simulink model "AssembledTEST1"  (R2016b)
settings: Solver=VariableStepAuto  StartTime=0.0  StopTime=60  RelTol=1e-9
values from neighbouring files (symbols this model uses):
  DOWN_0 = -xtrim(12)    [Comparison_NonLin.m]    (also in InitialiseJ31.m = 1830.0192; Trim.m)
  EAST_0 = xtrim(11)    [Comparison_NonLin.m]    (also in InitialiseJ31.m = 0; Trim.m)
  FLAP = 0    [InitialiseJ31.m]
  INERTIA = [IXX,IXY,IXZ;IXY,IYY,IYZ;IXZ,IYZ,IZZ]    [InitialiseJ31.m]
  NORTH_0 = xtrim(10)    [Comparison_NonLin.m]    (also in InitialiseJ31.m = 0; Trim.m)
  P_0 = xtrim(4)    [Comparison_NonLin.m]    (also in InitialiseJ31.m = 0; Trim.m)
  PHI_0 = xtrim(7)    [Comparison_NonLin.m]    (also in Trim.m)
  PSI_0 = xtrim(9)    [Comparison_NonLin.m]    (also in Trim.m)
  Q_0 = xtrim(5)    [Comparison_NonLin.m]    (also in InitialiseJ31.m = 0; Trim.m)
  R2D = 180/pi    (= 57.2957795131)    [InitialiseJ31.m]
  R_0 = xtrim(6)    [Comparison_NonLin.m]    (also in InitialiseJ31.m = 0; Trim.m)
  THETA_0 = xtrim(8)    [Comparison_NonLin.m]    (also in Trim.m)
  U_0 = xtrim(1)    [Comparison_NonLin.m]    (also in Trim.m)
  V_0 = xtrim(2)    [Comparison_NonLin.m]    (also in Trim.m)
  W_0 = xtrim(3)    [Comparison_NonLin.m]    (also in Trim.m)
undefined symbols (not defined in the file or in its folder): ail_data, Ap, Aw, b, beta0_data, c0, c_i, cdrag_data, CG, clean_wing_data, crt, CT_data, D, D0q_10, D0q_20, D0q_35, DCDi_data, DCM0b, Deh_f_on_data, Deh_on_data, df, Dqhq_data, e0, e_data10, e_data20, e_data35, elaw_0, elaw_1, elaw_2, flaps_lift_data, flaps_moment_data, flaps_tail_data, flaps_wing_data, fmc_data, fmf_data, fmn_data, fus_data, gamma_t, h_data10, h_data20, h_data35, it, iw, Iwn2, J_W, K1_data, k1f_data, k_data, L_r0_10f, L_r0_20f, L_r0_35f, l_t, ld_data, Lt, Lt_dash, Lv_b, Lv_h, Lv_n, mac, mach_ffr ... (+39)
libraries: aerolibasang x3, aerolibatmos2 x1
(part 1 of 5)
settings Model: Creator=pereantoni  LastModifiedBy=carles
settings SolverCC: ZeroCrossControl=DisableAll
settings DataIOCC: SaveFormat=Array

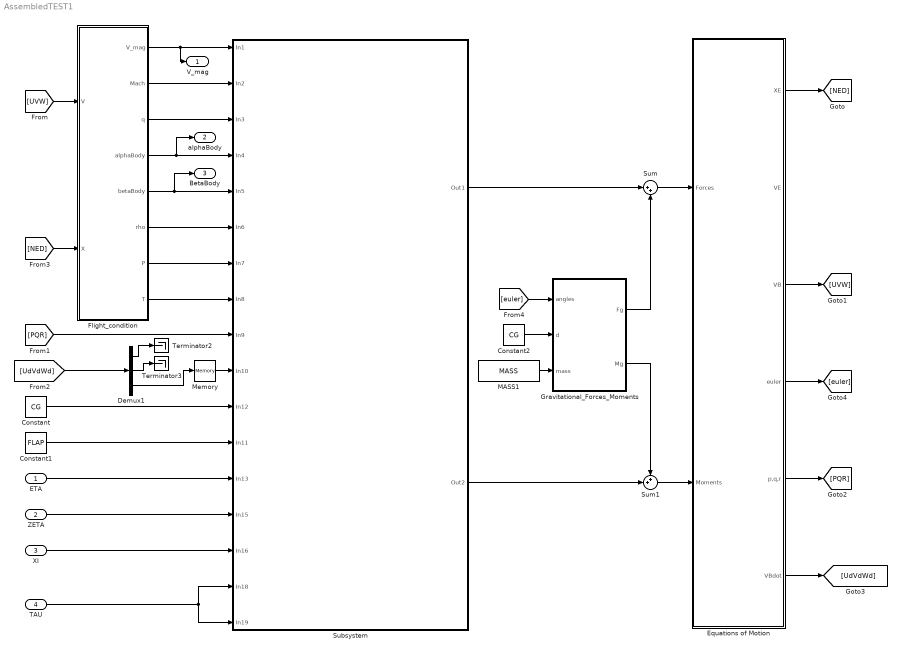
== system AssembledTEST1 ==
  ETA : Inport
  ZETA : Inport  Port=2
  XI : Inport  Port=3
  "TAU " : Inport  Port=4
  Constant : Constant  Value=CG
  Constant1 : Constant  Value=FLAP
  Constant2 : Constant  Value=CG
  Demux1 : Demux  Outputs=3
  Equations of Motion : Subsystem
  Flight_condition : Subsystem
  Gravitational_Forces_Moments : MATLAB Function  TreatAsAtomicUnit=on
  MASS1 : Constant  Value=MASS
  Memory : Memory
  Subsystem : Subsystem
      mask help:
      | This subsystem generates forces and moments about the body axes centre for a standard
      | Jetstream J31. The method of calculating the fuselage forces and moments has been
      | adjusted to reflect the latest issue of the J31 datapack.
      |
      | Completed by A Cooke - Jan 2010
      mask Display:
      | port_label('output',1,'F [N]')
      | port_label('output',2,'M [Nm]')
      | text(0.32,0.5,'Jetstream 31 Aircraft Model')
      | text(0.29,0.48,'Forces and Moments about BAC')
      | port_label('input',1,'V (m/s)')
      | port_label('input',2,'Mach')
      | port_label('input',3,'q_\infty (N/m^2)','texmode','on')
      | port_label('input',4,'\alpha (rad)','texmode','on')
      | port_label('input',5,'\beta (rad)','texmode','on')
      | port_label('input',6,'\rho (kg/m^3)','texmode','on')
      | port_label('input',7,'P (N/m^2)','texmode','on')
      | port_label('input',8,'T (K)','texmode','on')
      | port_label('input',9,'\omega (rad/s)','texmode','on')
      | port_label('input',10,'dw/dt (m/s^2)','texmode','on')
      | port_label('input',12,'Flap [0, 1, 2 or 3]')
      | port_label('input',11,'[xyz]_{cg} (m)','texmode','on')
      | port_label('input',13,'\eta (rad)','texmode','on')
      | port_label('input',14,'\zeta (rad)','texmode','on')
      | port_label('input',15,'\xi (rad)','texmode','on')
      | port_label('input',16,'\tau_L (%)','texmode','on')
      | port_label('input',17,'\tau_R (%)','texmode','on')
      | text(0.8,0.02,'\copyright AKC 2010','texmode','on')
      | text(0.23,0.99,'AERODYNAMIC & PROPULSIVE ONLY')
      | text(0.37,0.97,'Version 3 - 16 Jan 10')
  Sum : Sum  Inputs=|++
  Sum1 : Sum  Inputs=++|
  Terminator2 : Terminator
  Terminator3 : Terminator
  V_mag : Outport
  alphaBody : Outport  Port=2
  BetaBody : Outport  Port=3
  wires:
  Equations of Motion/1(XE) -> [NED]
  Subsystem/1(Out1) -> Sum/1
  Subsystem/2(Out2) -> Sum1/2
  Constant1/1 -> Subsystem/12(In11)
  [PQR] -> Subsystem/9(In9)
  Constant/1 -> Subsystem/11(In12)
  XI/1 -> Subsystem/15(In16)
  ZETA/1 -> Subsystem/14(In15)
  ETA/1 -> Subsystem/13(In13)
  Demux1/3 -> Memory/1
  Demux1/1 -> Terminator2/1
  Demux1/2 -> Terminator3/1
  Equations of Motion/3(VB) -> [UVW]
  Equations of Motion/4(euler) -> [euler]
  Equations of Motion/5(p,q,r) -> [PQR]
  Equations of Motion/6(VBdot) -> [UdVdWd]
  [UdVdWd] -> Demux1/1
  Memory/1 -> Subsystem/10(In10)
  "TAU "/1 -> Subsystem/16(In18), Subsystem/17(In19)
  Constant2/1 -> Gravitational_Forces_Moments/2(d)
  MASS1/1 -> Gravitational_Forces_Moments/3(mass)
  Sum/1 -> Equations of Motion/1(Forces)
  Gravitational_Forces_Moments/1(Fg) -> Sum/2
  Sum1/1 -> Equations of Motion/2(Moments)
  Gravitational_Forces_Moments/2(Mg) -> Sum1/1
  [euler] -> Gravitational_Forces_Moments/1(angles)
  Flight_condition/1(V_mag) -> V_mag/1, Subsystem/1(In1)
  [UVW] -> Flight_condition/1(V)
  [NED] -> Flight_condition/2(X)
  Flight_condition/2(Mach) -> Subsystem/2(In2)
  Flight_condition/3(q) -> Subsystem/3(In3)
  Flight_condition/4(alphaBody) -> alphaBody/1, Subsystem/4(In4)
  Flight_condition/5(betaBody) -> BetaBody/1, Subsystem/5(In5)
  Flight_condition/6(rho) -> Subsystem/6(In6)
  Flight_condition/7(P) -> Subsystem/7(In7)
  Flight_condition/8(T) -> Subsystem/8(In8)

== system AssembledTEST1/Equations of Motion ==
  Forces : Inport
  Moments : Inport  Port=2
  Constant : Constant  Value=CG
  EoMs : MATLAB Function  TreatAsAtomicUnit=on
  Gain : Gain  Gain=[1;1;-1]
  INERTIA A : Constant  Value=INERTIA
  MASS : Constant  Value=MASS
  Navigation_equations : Subsystem
  Rotational_Kinematic_Transform : MATLAB Function  TreatAsAtomicUnit=on
  V : Integrator  Tag='V'  Priority=1  InitialCondition=[U_0;V_0;W_0]  ContinuousStateAttributes='V'
  X : Integrator  Tag='X'  Priority=4  InitialCondition=[NORTH_0 EAST_0 -DOWN_0]  ContinuousStateAttributes='X'
  "p, q, r" : Integrator  Tag='omega'  Priority=2  InitialCondition=[P_0;Q_0;R_0]  ContinuousStateAttributes='omega'
  "phi, theta, psi" : Integrator  Tag='euler'  Priority=3  InitialCondition=[PHI_0;THETA_0;PSI_0]  ContinuousStateAttributes='euler'
  XE : Outport
  VE : Outport  Port=2
  VB : Outport  Port=3
  euler : Outport  Port=4
  p,q,r : Outport  Port=5
  VBdot : Outport  Port=6
  wires:
  INERTIA A/1 -> EoMs/6(INERTIA)
  MASS/1 -> EoMs/5(MASS)
  X/1 -> Gain/1
  V/1 -> Navigation_equations/1(VB), VB/1, EoMs/3(velocity)
  "p, q, r"/1 -> Rotational_Kinematic_Transform/2(rates), p,q,r/1, EoMs/4(omega)
  EoMs/1(Vdot) -> VBdot/1, V/1
  Constant/1 -> EoMs/7(CG)
  Forces/1 -> EoMs/1(Forces)
  Moments/1 -> EoMs/2(Moments)
  EoMs/2(omegadot) -> "p, q, r"/1
  Rotational_Kinematic_Transform/1(anglesDot) -> "phi, theta, psi"/1
  "phi, theta, psi"/1 -> euler/1, Navigation_equations/2(Attitude), Rotational_Kinematic_Transform/1(angles)
  Gain/1 -> XE/1
  Navigation_equations/1(VE) -> VE/1, X/1

== system AssembledTEST1/Flight_condition ==
  V : Inport
  X : Inport  Port=2
  Demux : Demux  Outputs=3
  Dynamic Pressure : aerolibasang/Dynamic Pressure
  ISA Atmosphere Model : aerolibatmos2/ISA Atmosphere Model  custom=on  g=9.80665  gamma=1.4  R=287.0531  L=0.0065  h_trop=11000  h_strat=20000  rho0=1.225  P0=101325  T0=288.15  h0=0
  "Incidence, Sideslip, & Airspeed" : aerolibasang/Incidence, Sideslip, & Airspeed
  Mach Number : aerolibasang/Mach Number
  Terminator : Terminator
  Terminator1 : Terminator
  V_mag : Outport
  Mach : Outport  Port=2
  q : Outport  Port=3
  alphaBody : Outport  Port=4
  betaBody : Outport  Port=5
  rho : Outport  Port=6
  P : Outport  Port=7
  T : Outport  Port=8
  wires:
  ISA Atmosphere Model/2 -> Mach Number/2
  "Incidence, Sideslip, & Airspeed"/3 -> V_mag/1
  "Incidence, Sideslip, & Airspeed"/2 -> betaBody/1
  Mach Number/1 -> Mach/1
  X/1 -> Demux/1
  ISA Atmosphere Model/1 -> T/1
  Demux/2 -> Terminator1/1
  Demux/3 -> ISA Atmosphere Model/1
  ISA Atmosphere Model/3 -> P/1
  Dynamic Pressure/1 -> q/1
  V/1 -> "Incidence, Sideslip, & Airspeed"/1, Mach Number/1, Dynamic Pressure/1
  Demux/1 -> Terminator/1
  "Incidence, Sideslip, & Airspeed"/1 -> alphaBody/1
  ISA Atmosphere Model/4 -> rho/1, Dynamic Pressure/2

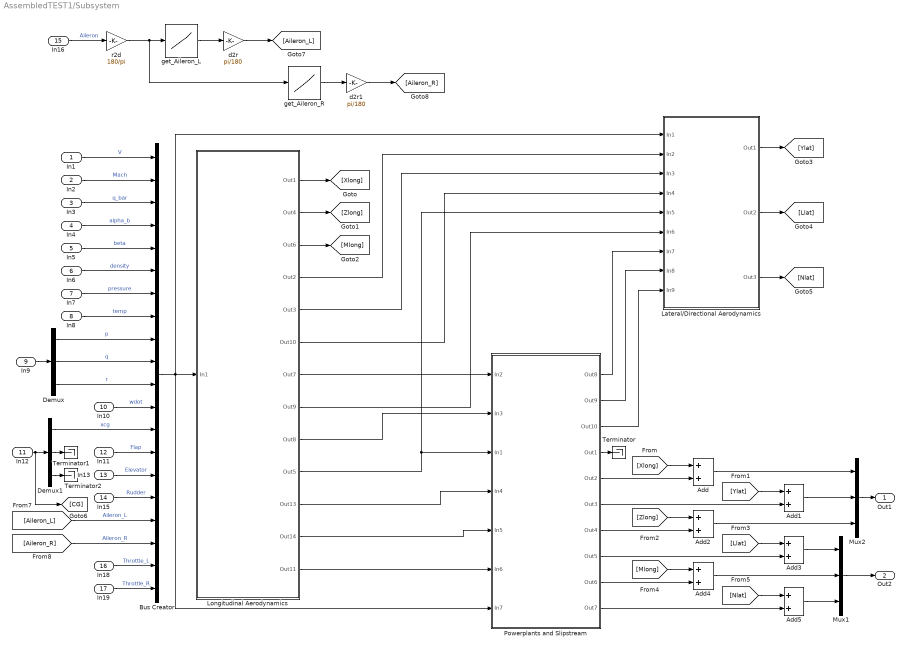
== system AssembledTEST1/Subsystem ==
  In1 : Inport
  In2 : Inport  Port=2
  In3 : Inport  Port=3
  In4 : Inport  Port=4
  In5 : Inport  Port=5
  In6 : Inport  Port=6
  In7 : Inport  Port=7
  In8 : Inport  Port=8
  In9 : Inport  Port=9
  In10 : Inport  Port=10
  In12 : Inport  Port=11
  In11 : Inport  Port=12
  In13 : Inport  Port=13
  In15 : Inport  Port=14
  In16 : Inport  Port=15
  In18 : Inport  Port=16
  In19 : Inport  Port=17
  Add{,1..5} (6 alike) : Sum
  Bus Creator : BusCreator  Inputs=20
  Demux : Demux  Outputs=3
  Demux1 : Demux  Outputs=3
  Lateral/Directional Aerodynamics : Subsystem
      mask Display:
      | port_label('input',1,'Input Bus')
      | port_label('input',4,'C_{D0w}','texmode','on')
      | port_label('input',2,'\DeltaC_{{Di}_{flap}}','texmode','on')
      | port_label('input',3,'\DeltaC_{{D0}_{flap}}','texmode','on')
      | port_label('input',5,'C_{Lw}','texmode','on')
      | port_label('input',6,'C_{Lb}','texmode','on')
      | port_label('input',7,'mean X_P [N]','texmode','on')
      | port_label('input',8,'mean \partial\epsilon_u/\partial\alpha_p','texmode','on')
      | port_label('output',1,'Y [N}')
      | port_label('output',2,'L [Nm]')
      | port_label('output',3,'N [Nm]')
      | port_label('input',9,'mean (\DeltaC_{Lw})_{slip}','texmode','on')
  Longitudinal Aerodynamics : Subsystem
      mask Display:
      | port_label('input',1,'Input Bus')
      | port_label('output',1,'X [N]')
      | port_label('output',2,'Z [N}')
      | port_label('output',3,'M [Nm]')
      | port_label('output',4,'\Delta C_{Di_{flap}}','texmode','on')
      | port_label('output',5,'\Delta C_{D0_{flap}}','texmode','on')
      | port_label('output',6,'C_{D0w}','texmode','on')
      | port_label('output',7,'a_{1t} [/rad]','texmode','on')
      | port_label('output',9,'\epsilon_h [rad]','texmode','on')
      | port_label('output',10,'C_{Lw}','texmode','on')
      | port_label('output',8,'C_{Lb}','texmode','on')
      | port_label('output',11,'C_{Lt}','texmode','on')
      | port_label('output',12,'\alpha_t [rad]','texmode','on')
      | port_label('output',13,'(C_{Dv})_W','texmode','on')
  Mux1 : Mux  Inputs=3
  Mux2 : Mux  Inputs=3
  Powerplants and Slipstream : Subsystem
      mask Display:
      | port_label('input',3,'C_{Lw}','texmode','on')
      | port_label('input',1,'a_{1t} [/rad]','texmode','on')
      | port_label('input',2,'\epsilon_h [rad]','texmode','on')
      | port_label('input',4,'C_{Lt}','texmode','on')
      | port_label('input',5,'\alpha_t [rad]','texmode','on')
      | port_label('input',6,'(C_{Dv})_W','texmode','on')
      | port_label('input',7,'Input Bus')
      | port_label('output',4,'FFR [kg/h]')
      | port_label('output',5,'X [N]')
      | port_label('output',6,'Y [N]')
      | port_label('output',7,'Z [N]')
      | port_label('output',8,'L [Nm]')
      | port_label('output',9,'M [Nm]')
      | port_label('output',10,'N [Nm]')
      | port_label('output',1,'mean X_P [N]','texmode','on')
      | port_label('output',2,'mean \partial\epsilon_u/\partial\alpha_p','texmode','on')
      | port_label('output',3,'mean (\DeltaC_{Lw})_{slip}','texmode','on')
  Terminator : Terminator
  Terminator1 : Terminator
  Terminator2 : Terminator
  d2r : Gain  Gain=pi/180
  d2r1 : Gain  Gain=pi/180
  get_Aileron_L : Lookup  InputValues=ail_data(1,:)  Table=ail_data(2,:)
  get_Aileron_R : Lookup  InputValues=ail_data(1,:)  Table=ail_data(3,:)
  r2d : Gain  Gain=180/pi
  Out1 : Outport
  Out2 : Outport  Port=2
  wires:
  Bus Creator/1 -> Longitudinal Aerodynamics/1(In1), Lateral/Directional Aerodynamics/1(In1), Powerplants and Slipstream/7(In7)
  Longitudinal Aerodynamics/4(Out2) -> Lateral/Directional Aerodynamics/2(In2)
  Longitudinal Aerodynamics/5(Out3) -> Lateral/Directional Aerodynamics/3(In3)
  Longitudinal Aerodynamics/6(Out10) -> Lateral/Directional Aerodynamics/4(In4)
  Longitudinal Aerodynamics/10(Out5) -> Lateral/Directional Aerodynamics/5(In5), Powerplants and Slipstream/3(In1)
  Longitudinal Aerodynamics/8(Out9) -> Lateral/Directional Aerodynamics/6(In6)
  Longitudinal Aerodynamics/11(Out13) -> Powerplants and Slipstream/4(In4)
  Longitudinal Aerodynamics/12(Out14) -> Powerplants and Slipstream/5(In5)
  Longitudinal Aerodynamics/7(Out7) -> Powerplants and Slipstream/1(In2)
  Longitudinal Aerodynamics/9(Out8) -> Powerplants and Slipstream/2(In3)
  Longitudinal Aerodynamics/13(Out11) -> Powerplants and Slipstream/6(In6)
  Demux/1 -> Bus Creator/9  "p"
  Demux/2 -> Bus Creator/10  "q"
  Demux/3 -> Bus Creator/11  "r"
  Demux1/1 -> Bus Creator/13  "xcg"
  Powerplants and Slipstream/4(Out1) -> Terminator/1
  Longitudinal Aerodynamics/1(Out1) -> [Xlong]
  Longitudinal Aerodynamics/2(Out4) -> [Zlong]
  Longitudinal Aerodynamics/3(Out6) -> [Mlong]
  Lateral/Directional Aerodynamics/1(Out1) -> [Ylat]
  Lateral/Directional Aerodynamics/2(Out2) -> [Llat]
  Lateral/Directional Aerodynamics/3(Out3) -> [Nlat]
  Powerplants and Slipstream/5(Out2) -> Add/2
  [Xlong] -> Add/1
  Powerplants and Slipstream/6(Out3) -> Add1/2
  [Ylat] -> Add1/1
  Powerplants and Slipstream/7(Out4) -> Add2/2
  [Zlong] -> Add2/1
  Powerplants and Slipstream/8(Out5) -> Add3/2
  [Llat] -> Add3/1
  Powerplants and Slipstream/9(Out6) -> Add4/2
  [Mlong] -> Add4/1
  Powerplants and Slipstream/10(Out7) -> Add5/2
  [Nlat] -> Add5/1
  Add/1 -> Mux2/1
  Add1/1 -> Mux2/2
  Add2/1 -> Mux2/3
  Add3/1 -> Mux1/1
  Add4/1 -> Mux1/2
  Add5/1 -> Mux1/3
  Mux1/1 -> Out2/1
  Demux1/2 -> Terminator1/1
  Demux1/3 -> Terminator2/1
  In1/1 -> Bus Creator/1  "V"
  In2/1 -> Bus Creator/2  "Mach"
  In3/1 -> Bus Creator/3  "q_bar"
  In4/1 -> Bus Creator/4  "alpha_b"
  In5/1 -> Bus Creator/5  "beta"
  In6/1 -> Bus Creator/6  "density"
  In7/1 -> Bus Creator/7  "pressure"
  In8/1 -> Bus Creator/8  "temp"
  Mux2/1 -> Out1/1
  In9/1 -> Demux/1
  In10/1 -> Bus Creator/12  "wdot"
  In11/1 -> Bus Creator/14  "Flap"
  In12/1 -> Demux1/1, [CG]
  In13/1 -> Bus Creator/15  "Elevator"
  In15/1 -> Bus Creator/16  "Rudder"
  In18/1 -> Bus Creator/19  "Throttle_L"
  In19/1 -> Bus Creator/20  "Throttle_R"
  In16/1 -> r2d/1  "Aileron"
  r2d/1 -> get_Aileron_L/1, get_Aileron_R/1
  [Aileron_L] -> Bus Creator/17  "Aileron_L"
  get_Aileron_L/1 -> d2r/1
  d2r/1 -> [Aileron_L]
  d2r1/1 -> [Aileron_R]
  get_Aileron_R/1 -> d2r1/1
  [Aileron_R] -> Bus Creator/18  "Aileron_R"
  Powerplants and Slipstream/1(Out8) -> Lateral/Directional Aerodynamics/7(In7)
  Powerplants and Slipstream/2(Out9) -> Lateral/Directional Aerodynamics/8(In8)
  Powerplants and Slipstream/3(Out10) -> Lateral/Directional Aerodynamics/9(In9)

== system AssembledTEST1/Equations of Motion/Navigation_equations ==
  VB : Inport
  Attitude : Inport  Port=2
  DCM_matrix : MATLAB Function  TreatAsAtomicUnit=on
  Divide : Product  Inputs=/  Multiplication=Matrix(*)
  Product1 : Product  Multiplication=Matrix(*)
  VE : Outport
  wires:
  Attitude/1 -> DCM_matrix/1(EUL)
  VB/1 -> Product1/2
  DCM_matrix/1(T) -> Divide/1
  Product1/1 -> VE/1
  Divide/1 -> Product1/1

== system AssembledTEST1/Subsystem/Lateral//Directional Aerodynamics ==
  In1 : Inport
  In2 : Inport  Port=2
  In3 : Inport  Port=3
  In4 : Inport  Port=4
  In5 : Inport  Port=5
  In6 : Inport  Port=6
  In7 : Inport  Port=7
  In8 : Inport  Port=8
  In9 : Inport  Port=9
  Bus Selector : BusSelector  OutputSignals=Mach,Flap,alpha_b,beta,q_bar,V,Aileron_L,Aileron_R,p,r,Rudder
  getYLN : Subsystem
      mask Display:
      | port_label('output',1,'Y')
      | port_label('output',2,'L')
      | port_label('output',3,'N')
      | port_label('input',1,'Mach')
      | port_label('input',2,'Flap')
      | port_label('input',3,'\alpha_b','texmode','on')
      | port_label('input',4,'\beta','texmode','on')
      | port_label('input',5,'0.5\rhoV^2 [N/m^2]','texmode','on')
      | port_label('input',6,'V')
      | port_label('input',7,'\xi_L','texmode','on')
      | port_label('input',8,'\xi_R','texmode','on')
      | port_label('input',15,'C_{Lw}','texmode','on')
      | port_label('input',16,'C_{Lb}','texmode','on')
      | port_label('input',9,'p')
      | port_label('input',10,'r')
      | port_label('input',11','\zeta','texmode','on')
      | port_label('input',14,'C_{D0w}','texmode','on')
      | port_label('input',12,'\DeltaC_{{Di}_{flap}}','texmode','on')
      | port_label('input',13,'\DeltaC_{{D0}_{flap}}','texmode','on')
      | text(0.2,0.5,'lateral/directional aerodynamics')
      | port_label('input',17,'mean X_P [N]','texmode','on')
      | port_label('input',18,'mean \partial\epsilon_u/\partial\alpha_p','texmode','on')
      | port_label('input',19,'mean (\DeltaC_{Lw})_{slip}','texmode','on')
  Out1 : Outport
  Out2 : Outport  Port=2
  Out3 : Outport  Port=3
  wires:
  Bus Selector/1 -> getYLN/1(In1)  "<Mach>"
  Bus Selector/2 -> getYLN/2(In13)  "<Flap>"
  Bus Selector/3 -> getYLN/3(In2)  "<alpha_b>"
  Bus Selector/4 -> getYLN/4(In3)  "<beta>"
  Bus Selector/5 -> getYLN/5(In4)  "<q_bar>"
  Bus Selector/6 -> getYLN/6(In5)  "<V>"
  Bus Selector/7 -> getYLN/7(In6)  "<Aileron_L>"
  Bus Selector/8 -> getYLN/8(In7)  "<Aileron_R>"
  Bus Selector/9 -> getYLN/9(In10)  "<p>"
  Bus Selector/10 -> getYLN/10(In11)  "<r>"
  Bus Selector/11 -> getYLN/11(In12)  "<Rudder>"
  In1/1 -> Bus Selector/1
  getYLN/1(Out1) -> Out1/1
  getYLN/2(Out2) -> Out2/1
  In2/1 -> getYLN/12(In15)
  In3/1 -> getYLN/13(In16)
  In4/1 -> getYLN/14(In14)
  getYLN/3(Out3) -> Out3/1
  In5/1 -> getYLN/15(In8)
  In6/1 -> getYLN/16(In9)
  In7/1 -> getYLN/17(In17)
  In8/1 -> getYLN/18(In18)
  In9/1 -> getYLN/19(In19)

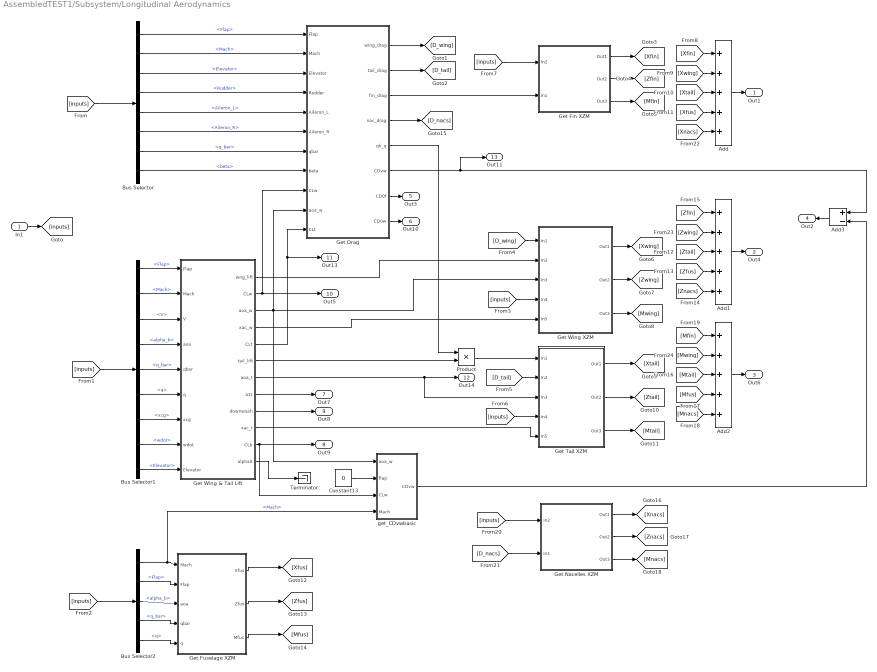
== system AssembledTEST1/Subsystem/Longitudinal Aerodynamics ==
  In1 : Inport
  Add : Sum  Inputs=+++++
  Add1 : Sum  Inputs=+++++
  Add2 : Sum  Inputs=+++++
  Add3 : Sum  Inputs=+-
  Bus Selector : BusSelector  OutputSignals=Flap,Mach,Elevator,Rudder,Aileron_L,Aileron_R,q_bar,beta
  Bus Selector1 : BusSelector  OutputSignals=Flap,Mach,V,alpha_b,q_bar,q,xcg,wdot,Elevator
  Bus Selector2 : BusSelector  OutputSignals=Mach,Flap,alpha_b,q_bar,q
  Constant13 : Constant  Value=0
  Get Drag : Subsystem
      mask Display:
      | port_label('output',1,'D_{wing} [N]','texmode','on')
      | port_label('output',2,'D_{tail} [N]','texmode','on')
      | port_label('output',3,'D_{fin} [N]','texmode','on')
      | port_label('output',4,'D_{nacs} [N]','texmode','on')
      | port_label('output',5,'q_h/q_\infty','texmode','on')
      | port_label('output',6,'(C_{Di})_w','texmode','on')
      | port_label('output',7,'\DeltaC_{D0_{flap}}','texmode','on')
      | port_label('output',8,'C_{D0w}','texmode','on')
      | port_label('input',1,'Flap')
      | port_label('input',2,'Mach')
      | port_label('input',3,'Elevator [rad]')
      | port_label('input',4,'Rudder [rad]')
      | port_label('input',5,'Left Aileron [rad]')
      | port_label('input',6,'Right Aileron [rad]')
      | port_label('input',7,'0.5\rhoV^2 [N/m^2]','texmode','on')
      | port_label('input',9,'C_{Lw}','texmode','on')
      | port_label('input',10,'\alpha_w [rad]','texmode','on')
      | port_label('input',11,'C_{Lt}','texmode','on')
      | port_label('input',8,'\beta [rad]','texmode','on')
  Get Fin XZM : Subsystem
      mask Display:
      | port_label('output',1,'X_{fin} [N]','texmode','on')
      | port_label('output',2,'Z_{fin} [N]','texmode','on')
      | port_label('output',3,'M_{fin} [Nm]','texmode','on')
      | port_label('input',2,'D_{fin} [N]','texmode','on')
  Get Fuselage XZM : Subsystem
      mask Display:
      | port_label('output',1,'X_{fus} [N]','texmode','on')
      | port_label('output',2,'Z_{fus} [N]','texmode','on')
      | port_label('output',3,'M_{fus} [Nm]','texmode','on')
      | port_label('input',2,'Flap')
      | port_label('input',1,'Mach')
      | port_label('input',3,'\alpha_{b} [rad]','texmode','on')
      | port_label('input',4,'0.5\rhoV^2 [N/m^2]','texmode','on')
      | port_label('input',5,'q [rad/s]')
  Get Nacelles XZM : Subsystem
      mask Display:
      | port_label('output',1,'X_{nacs} [N]','texmode','on')
      | port_label('output',2,'Z_{nacs} [N]','texmode','on')
      | port_label('output',3,'M_{nacs} [Nm]','texmode','on')
      | port_label('input',2,'D_{nacs} [N]','texmode','on')
  Get Tail XZM : Subsystem
      mask Display:
      | port_label('output',1,'X_{tail} [N]','texmode','on')
      | port_label('output',2,'Z_{tail} [N]','texmode','on')
      | port_label('output',3,'M_{tail} [Nm]','texmode','on')
      | port_label('input',1,'L_{tail} [N]','texmode','on')
      | port_label('input',3,'\alpha_{t} [rad]','texmode','on')
      | port_label('input',5,'x_{act} [m]','texmode','on')
  Get Wing & Tail Lift : Subsystem
      mask Display:
      | port_label('input',1,'Flap')
      | port_label('input',2,'Mach')
      | port_label('input',3,'V [m/s]')
      | port_label('input',4,'\alpha_b [rad]','texmode','on')
      | port_label('input',5,'0.5\rhoV^2 [N/m^2]','texmode','on')
      | port_label('input',6,'q [rad/s]')
      | port_label('input',7,'x_{cg} [m]','texmode','on')
      | port_label('input',8,'dw/dt')
      | port_label('input',9,'Elevator [rad]')
      | port_label('output',1,'L_{wing} [N]','texmode','on')
      | port_label('output',2,'C_{Lw}','texmode','on')
      | port_label('output',3,'\alpha_w [rad]','texmode','on')
      | port_label('output',4,'x_{acw} [m]','texmode','on')
      | port_label('output',7,'\alpha_t [rad]','texmode','on')
      | port_label('output',5,'C_{Lt}','texmode','on')
      | port_label('output',6,'L_{tail} [N]','texmode','on')
      | port_label('output',8,'a_{1t} [/rad]','texmode','on')
      | port_label('output',9,'\epsilon_h [rad]','texmode','on')
      | port_label('output',10,'x_{act} [m]','texmode','on')
      | port_label('output',11,'C_{Lb}','texmode','on')
      | port_label('output',12,'\alpha_0','texmode','on')
  Get Wing XZM : Subsystem
      mask Display:
      | port_label('output',1,'X_{wing} [N]','texmode','on')
      | port_label('output',2,'Z_{wing} [N]','texmode','on')
      | port_label('output',3,'M_{wing} [Nm]','texmode','on')
      | port_label('input',2,'L_{wing} [N]','texmode','on')
      | port_label('input',3,'\alpha_{w} [rad]','texmode','on')
      | port_label('input',5,'x_{acw} [m]','texmode','on')
  Product : Product  RndMeth=Zero
  Terminator : Terminator
  get_CDvwbasic : Subsystem
  Out1 : Outport
  Out4 : Outport  Port=2
  Out6 : Outport  Port=3
  Out2 : Outport  Port=4
  Out3 : Outport  Port=5
  Out10 : Outport  Port=6
  Out7 : Outport  Port=7
  Out9 : Outport  Port=8
  Out8 : Outport  Port=9
  Out5 : Outport  Port=10
  Out13 : Outport  Port=11
  Out14 : Outport  Port=12
  Out11 : Outport  Port=13
  wires:
  Get Wing & Tail Lift/1(wng_lift) -> Get Wing XZM/2(In2)
  Get Wing & Tail Lift/2(CLw) -> Get Drag/9(CLw), Out5/1
  Get Wing & Tail Lift/3(aoa_w) -> Get Drag/10(aoa_w), Get Wing XZM/3(In3), get_CDvwbasic/1(aoa_w)
  Get Wing & Tail Lift/4(xac_w) -> Get Wing XZM/5(In5)
  Get Fuselage XZM/1(Xfus) -> [Xfus]
  Get Fuselage XZM/2(Zfus) -> [Zfus]
  Get Fuselage XZM/3(Mfus) -> [Mfus]
  Get Wing & Tail Lift/5(CLt) -> Get Drag/11(CLt), Out13/1
  Bus Selector/1 -> Get Drag/1(Flap)  "<Flap>"
  Bus Selector/2 -> Get Drag/2(Mach)  "<Mach>"
  Bus Selector/3 -> Get Drag/3(Elevator)  "<Elevator>"
  Bus Selector/4 -> Get Drag/4(Rudder)  "<Rudder>"
  Bus Selector/5 -> Get Drag/5(Aileron_L)  "<Aileron_L>"
  Bus Selector/6 -> Get Drag/6(Aileron_R)  "<Aileron_R>"
  Bus Selector/7 -> Get Drag/7(qbar)  "<q_bar>"
  Bus Selector1/1 -> Get Wing & Tail Lift/1(Flap)  "<Flap>"
  Bus Selector1/2 -> Get Wing & Tail Lift/2(Mach)  "<Mach>"
  Bus Selector1/3 -> Get Wing & Tail Lift/3(V)  "<V>"
  Bus Selector1/4 -> Get Wing & Tail Lift/4(aoa)  "<alpha_b>"
  Bus Selector1/5 -> Get Wing & Tail Lift/5(qbar)  "<q_bar>"
  Bus Selector1/6 -> Get Wing & Tail Lift/6(q)  "<q>"
  Bus Selector1/7 -> Get Wing & Tail Lift/7(xcg)  "<xcg>"
  Bus Selector1/8 -> Get Wing & Tail Lift/8(wdot)  "<wdot>"
  Bus Selector1/9 -> Get Wing & Tail Lift/9(Elevator)  "<Elevator>"
  Bus Selector2/1 -> get_CDvwbasic/4(Mach), Get Fuselage XZM/1(Mach)  "<Mach>"
  [inputs] -> Bus Selector/1
  [inputs] -> Bus Selector1/1
  [inputs] -> Bus Selector2/1
  [inputs] -> Get Wing XZM/4(In4)
  Get Drag/1(wing_drag) -> [D_wing]
  [D_wing] -> Get Wing XZM/1(In1)
  Bus Selector/8 -> Get Drag/8(beta)  "<beta>"
  Get Drag/2(tail_drag) -> [D_tail]
  Get Wing & Tail Lift/7(aoa_t) -> Get Tail XZM/3(In3), Out14/1
  Get Wing & Tail Lift/10(xac_t) -> Get Tail XZM/5(In5)
  [D_tail] -> Get Tail XZM/2(In2)
  [inputs] -> Get Tail XZM/4(In4)
  Get Drag/3(fin_drag) -> Get Fin XZM/2(In1)
  [inputs] -> Get Fin XZM/1(In2)
  Get Fin XZM/1(Out1) -> [Xfin]
  Get Fin XZM/2(Out2) -> [Zfin]
  Get Fin XZM/3(Out3) -> [Mfin]
  Get Wing XZM/1(Out1) -> [Xwing]
  Get Wing XZM/2(Out2) -> [Zwing]
  Get Wing XZM/3(Out3) -> [Mwing]
  Get Tail XZM/1(Out1) -> [Xtail]
  Get Tail XZM/2(Out2) -> [Ztail]
  Get Tail XZM/3(Out3) -> [Mtail]
  [Xfin] -> Add/1
  [Xwing] -> Add/2
  [Xtail] -> Add/3
  [Xfus] -> Add/4
  Get Drag/4(nac_drag) -> [D_nacs]
  [inputs] -> Get Nacelles XZM/1(In2)
  Get Nacelles XZM/1(Out1) -> [Xnacs]
  Get Nacelles XZM/2(Out2) -> [Znacs]
  Get Nacelles XZM/3(Out3) -> [Mnacs]
  [D_nacs] -> Get Nacelles XZM/2(In1)
  [Xnacs] -> Add/5
  [Zfin] -> Add1/1
  [Zwing] -> Add1/2
  [Ztail] -> Add1/3
  [Zfus] -> Add1/4
  [Znacs] -> Add1/5
  [Mfin] -> Add2/1
  [Mwing] -> Add2/2
  [Mtail] -> Add2/3
  [Mfus] -> Add2/4
  [Mnacs] -> Add2/5
  Product/1 -> Get Tail XZM/1(In1)
  Get Wing & Tail Lift/6(tail_lift) -> Product/2
  Get Drag/5(qh_q) -> Product/1
  Get Drag/6(CDvw) -> Add3/1, Out11/1
  Get Wing & Tail Lift/11(CLb) -> get_CDvwbasic/3(CLw), Out9/1
  Constant13/1 -> get_CDvwbasic/2(flap)
  get_CDvwbasic/1(CDvw) -> Add3/2
  Add/1 -> Out1/1
  Add3/1 -> Out2/1
  Get Drag/7(CD0f) -> Out3/1
  In1/1 -> [inputs]
  Add1/1 -> Out4/1
  Add2/1 -> Out6/1
  Get Wing & Tail Lift/8(a1t) -> Out7/1
  Get Wing & Tail Lift/9(downwash) -> Out8/1
  Get Drag/8(CD0w) -> Out10/1
  Bus Selector2/2 -> Get Fuselage XZM/2(Flap)  "<Flap>"
  Bus Selector2/3 -> Get Fuselage XZM/3(aoa)  "<alpha_b>"
  Bus Selector2/4 -> Get Fuselage XZM/4(qbar)  "<q_bar>"
  Bus Selector2/5 -> Get Fuselage XZM/5(q)  "<q>"
  Get Wing & Tail Lift/12(alpha0) -> Terminator/1

== system AssembledTEST1/Subsystem/Powerplants and Slipstream ==
  In2 : Inport
  In3 : Inport  Port=2
  In1 : Inport  Port=3
  In4 : Inport  Port=4
  In5 : Inport  Port=5
  In6 : Inport  Port=6
  In7 : Inport  Port=7
  Bus Selector : BusSelector  OutputSignals=density,V,pressure,temp,Flap,Mach,alpha_b,beta,p,q,r,Elevator,Throttle_L,Throttle_R
  Subsystem2 : Subsystem
      mask Display:
      | port_label('output',1,'FFR [kg/h]')
      | text(0.4,0.5,'Powerplant Model')
      | text(0.35,0.01,'(includes slipstream effects)')
      | port_label('input',10,'P_\infty [N/m^2]','texmode','on')
      | port_label('input',8,'\rho_\infty [kg/m^3]','texmode','on')
      | port_label('input',11,'T_\infty [K]','texmode','on')
      | port_label('input',12,'Flap')
      | port_label('input',9,'V [m/s]')
      | port_label('input',14,'\alpha_b [rad]','texmode','on')
      | port_label('input',15,'\beta [rad]','texmode','on')
      | port_label('input',16,'p [rad/s]')
      | port_label('input',17,'q [rad/s]')
      | port_label('input',18,'r [rad/s]')
      | port_label('input',13,'Mach')
      | port_label('input',1,'C_{Lw}','texmode','on')
      | port_label('input',20,'Left Throttle [%]')
      | port_label('input',21,'Right Throttle [%]')
      | port_label('input',3,'\epsilon_h [rad]','texmode','on')
      | port_label('input',7,'(C_{M0})_w','texmode','on')
      | port_label('input',6,'(C_{Dv})_w','texmode','on')
      | port_label('input',4,'C_{Lt}','texmode','on')
      | port_label('input',2,'a_{1t} [/rad]','texmode','on')
      | port_label('input',19,'Elevator [rad]')
      | port_label('input',5,'\alpha_{t} [rad]','texmode','on')
      | port_label('output',2,'X [N]')
      | port_label('output',3,'Y [N]')
      | port_label('output',4,'Z [N]')
      | port_label('output',5,'L [Nm]')
      | port_label('output',6,'M [Nm]')
      | port_label('output',7,'N [Nm]')
      | port_label('output',8,'mean X_P [N]','texmode','on')
      | port_label('output',9,'mean \partial\epsilon_u/\partial\alpha_p','texmode','on')
      | port_label('output',10,'mean (\DeltaC_{Lw})_{slip}','texmode','on')
  get_CM0 : Subsystem
  Out8 : Outport
  Out9 : Outport  Port=2
  Out10 : Outport  Port=3
  Out1 : Outport  Port=4
  Out2 : Outport  Port=5
  Out3 : Outport  Port=6
  Out4 : Outport  Port=7
  Out5 : Outport  Port=8
  Out6 : Outport  Port=9
  Out7 : Outport  Port=10
  wires:
  get_CM0/1(CM0) -> Subsystem2/7(In8)
  Bus Selector/1 -> Subsystem2/8(In1)  "<density>"
  Bus Selector/2 -> Subsystem2/9(In2)  "<V>"
  Bus Selector/3 -> Subsystem2/10(In3)  "<pressure>"
  Bus Selector/4 -> Subsystem2/11(In4)  "<temp>"
  Bus Selector/5 -> get_CM0/2(Flap), Subsystem2/12(In5)  "<Flap>"
  Bus Selector/6 -> Subsystem2/13(In6), get_CM0/1(Mach)  "<Mach>"
  Bus Selector/7 -> Subsystem2/14(In7)  "<alpha_b>"
  Bus Selector/8 -> Subsystem2/15(In9)  "<beta>"
  Bus Selector/9 -> Subsystem2/16(In11)  "<p>"
  Bus Selector/10 -> Subsystem2/17(In12)  "<q>"
  Bus Selector/11 -> Subsystem2/18(In10)  "<r>"
  Bus Selector/12 -> Subsystem2/19(In19)  "<Elevator>"
  Bus Selector/13 -> Subsystem2/20(In13)  "<Throttle_L>"
  Bus Selector/14 -> Subsystem2/21(In21)  "<Throttle_R>"
  In7/1 -> Bus Selector/1
  In2/1 -> Subsystem2/2(In18)
  Subsystem2/1(Out4) -> Out1/1
  In3/1 -> Subsystem2/3(In15)
  In4/1 -> Subsystem2/4(In17)
  In5/1 -> Subsystem2/5(In20)
  In6/1 -> Subsystem2/6(In16)
  In1/1 -> Subsystem2/1(In14)
  Subsystem2/3(Out6) -> Out3/1
  Subsystem2/4(Out7) -> Out4/1
  Subsystem2/6(Out2) -> Out6/1
  Subsystem2/7(Out3) -> Out7/1
  Subsystem2/8(Out8) -> Out8/1
  Subsystem2/9(Out9) -> Out9/1
  Subsystem2/10(Out10) -> Out10/1
  Subsystem2/2(Out5) -> Out2/1
  Subsystem2/5(Out1) -> Out5/1

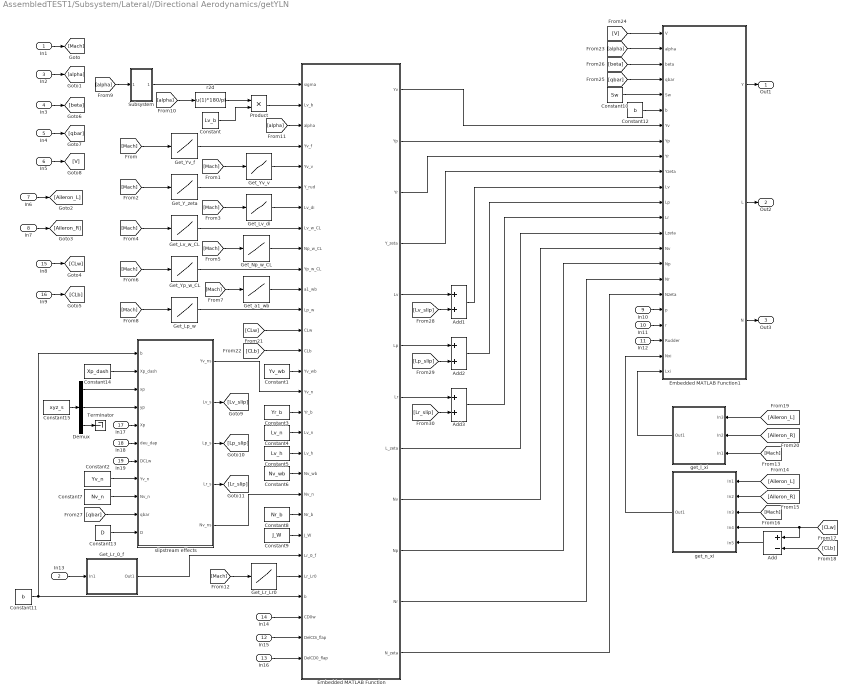
== system AssembledTEST1/Subsystem/Lateral//Directional Aerodynamics/getYLN ==
  In1 : Inport
  In13 : Inport  Port=2
  In2 : Inport  Port=3
  In3 : Inport  Port=4
  In4 : Inport  Port=5
  In5 : Inport  Port=6
  In6 : Inport  Port=7
  In7 : Inport  Port=8
  In10 : Inport  Port=9
  In11 : Inport  Port=10
  In12 : Inport  Port=11
  In15 : Inport  Port=12
  In16 : Inport  Port=13
  In14 : Inport  Port=14
  In8 : Inport  Port=15
  In9 : Inport  Port=16
  In17 : Inport  Port=17
  In18 : Inport  Port=18
  In19 : Inport  Port=19
  Add : Sum  Inputs=+-
  Add1 : Sum
  Add2 : Sum
  Add3 : Sum
  Constant : Constant  Value=Lv_b
  Constant1 : Constant  Value=Yv_wb
  Constant10 : Constant  Value=Sw
  Constant11 : Constant  Value=b
  Constant12 : Constant  Value=b
  Constant13 : Constant  Value=D
  Constant14 : Constant  Value=Xp_dash
  Constant15 : Constant  Value=xyz_s
  Constant2 : Constant  Value=Yv_n
  Constant3 : Constant  Value=Yr_b
  Constant4 : Constant  Value=Lv_n
  Constant5 : Constant  Value=Lv_h
  Constant6 : Constant  Value=Nv_wb
  Constant7 : Constant  Value=Nv_n
  Constant8 : Constant  Value=Nr_b
  Constant9 : Constant  Value=J_W
  Demux : Demux  Outputs=3
  Embedded MATLAB Function : MATLAB Function  TreatAsAtomicUnit=on
  Embedded MATLAB Function1 : MATLAB Function  TreatAsAtomicUnit=on
  Get_Lp_w : Lookup  InputValues=ld_data(:,1)  Table=ld_data(:,9)
  Get_Lr_0_f : Subsystem
      mask Display: port_label('input',1,'flap')
  Get_Lr_Lr0 : Lookup  InputValues=ld_data(:,1)  Table=ld_data(:,11)
  Get_Lv_di : Lookup  InputValues=ld_data(:,1)  Table=ld_data(:,4)
  Get_Lv_w_CL : Lookup  InputValues=ld_data(:,1)  Table=ld_data(:,5)
  Get_Np_w_CL : Lookup  InputValues=ld_data(:,1)  Table=ld_data(:,6)
  Get_Y_zeta : Lookup  InputValues=ld_data(:,1)  Table=ld_data(:,3)
  Get_Yp_w_CL : Lookup  InputValues=ld_data(:,1)  Table=ld_data(:,7)
  Get_Yv_f : Lookup  InputValues=ld_data(:,1)  Table=ld_data(:,2)
  Get_Yv_v : Lookup  InputValues=ld_data(:,1)  Table=ld_data(:,10)
  Get_a1_wb : Lookup  InputValues=ld_data(:,1)  Table=ld_data(:,8)
  Product : Product  RndMeth=Zero
  Subsystem : Subsystem
      mask Display:
      | port_label('input',1,'\alpha','texmode','on')
      | port_label('output',1,'\sigma','texmode','on')
  Terminator : Terminator
  get_l_xi : Subsystem
      mask Display:
      | port_label('input',1,'Aileron_L')
      | port_label('input',2,'Aileron_R')
      | port_label('input',3,'Mach')
      | port_label('output',1,'l_{\xi}','texmode','on')
  get_n_xi : Subsystem
      mask Display:
      | port_label('input',1,'Aileron_L')
      | port_label('input',2,'Aileron_R')
      | port_label('input',3,'Mach')
      | port_label('input',4,'C_{Lw}','texmode','on')
      | port_label('input',5,'\DeltaC_{flap}','texmode','on')
      | port_label('output',1,'n_{\xi}','texmode','on')
  r2d : Fcn  Expr=u(1)*180/pi
  slipstream effects : MATLAB Function  TreatAsAtomicUnit=on
  Out1 : Outport
  Out2 : Outport  Port=2
  Out3 : Outport  Port=3
  wires:
  [Mach] -> Get_Yv_f/1
  [Mach] -> Get_Yv_v/1
  [Mach] -> Get_Y_zeta/1
  [Mach] -> Get_Lv_di/1
  [Mach] -> Get_Lv_w_CL/1
  [Mach] -> Get_Np_w_CL/1
  [Mach] -> Get_Yp_w_CL/1
  [Mach] -> Get_a1_wb/1
  [Mach] -> Get_Lp_w/1
  [alpha] -> Subsystem/1(In1)
  Subsystem/1(Out1) -> Embedded MATLAB Function/1(sigma)
  [alpha] -> r2d/1
  r2d/1 -> Product/1
  Constant/1 -> Product/2
  Product/1 -> Embedded MATLAB Function/2(Lv_b)
  [alpha] -> Embedded MATLAB Function/3(alpha)
  Get_Yv_f/1 -> Embedded MATLAB Function/4(Yv_f)
  Get_Yv_v/1 -> Embedded MATLAB Function/5(Yv_v)
  Get_Lv_di/1 -> Embedded MATLAB Function/7(Lv_di)
  Get_Lv_w_CL/1 -> Embedded MATLAB Function/8(Lv_w_CL)
  Get_Np_w_CL/1 -> Embedded MATLAB Function/9(Np_w_CL)
  Get_Yp_w_CL/1 -> Embedded MATLAB Function/10(Yp_w_CL)
  Get_a1_wb/1 -> Embedded MATLAB Function/11(a1_wb)
  Get_Lp_w/1 -> Embedded MATLAB Function/12(Lp_w)
  Constant1/1 -> Embedded MATLAB Function/15(Yv_wb)
  Constant5/1 -> Embedded MATLAB Function/19(Lv_h)
  Constant3/1 -> Embedded MATLAB Function/17(Yr_b)
  Constant4/1 -> Embedded MATLAB Function/18(Lv_n)
  Constant6/1 -> Embedded MATLAB Function/20(Nv_wb)
  Constant8/1 -> Embedded MATLAB Function/22(Nr_b)
  Constant9/1 -> Embedded MATLAB Function/23(J_W)
  Get_Lr_0_f/1(Out1) -> Embedded MATLAB Function/24(Lr_0_f)
  [Mach] -> Get_Lr_Lr0/1
  Get_Lr_Lr0/1 -> Embedded MATLAB Function/25(Lr_Lr0)
  [Mach] -> get_l_xi/3(In1)
  [Aileron_L] -> get_n_xi/1(In1)
  [Aileron_R] -> get_n_xi/2(In2)
  [Mach] -> get_n_xi/3(In3)
  [CLw] -> get_n_xi/4(In4), Add/1
  Add/1 -> get_n_xi/5(In5)
  [CLb] -> Add/2
  [Aileron_R] -> get_l_xi/2(In2)
  [Aileron_L] -> get_l_xi/1(In3)
  [CLw] -> Embedded MATLAB Function/13(CLw)
  [CLb] -> Embedded MATLAB Function/14(CLb)
  Get_Y_zeta/1 -> Embedded MATLAB Function/6(Y_rud)
  Constant11/1 -> Embedded MATLAB Function/26(b), slipstream effects/1(b)
  Embedded MATLAB Function/1(Yv) -> Embedded MATLAB Function1/7(Yv)
  Embedded MATLAB Function/2(Yp) -> Embedded MATLAB Function1/8(Yp)
  Embedded MATLAB Function/3(Yr) -> Embedded MATLAB Function1/9(Yr)
  Embedded MATLAB Function/4(Y_zeta) -> Embedded MATLAB Function1/10(Yzeta)
  Constant10/1 -> Embedded MATLAB Function1/5(Sw)
  Constant12/1 -> Embedded MATLAB Function1/6(b)
  [alpha] -> Embedded MATLAB Function1/2(alpha)
  [V] -> Embedded MATLAB Function1/1(V)
  [qbar] -> Embedded MATLAB Function1/4(qbar)
  [beta] -> Embedded MATLAB Function1/3(beta)
  Embedded MATLAB Function/8(L_zeta) -> Embedded MATLAB Function1/14(Lzeta)
  get_l_xi/1(Out1) -> Embedded MATLAB Function1/23(Lxi)
  Embedded MATLAB Function/9(Nv) -> Embedded MATLAB Function1/15(Nv)
  Embedded MATLAB Function/10(Np) -> Embedded MATLAB Function1/16(Np)
  Embedded MATLAB Function/11(Nr) -> Embedded MATLAB Function1/17(Nr)
  Embedded MATLAB Function/12(N_zeta) -> Embedded MATLAB Function1/18(Nzeta)
  In1/1 -> [Mach]
  In2/1 -> [alpha]
  Embedded MATLAB Function1/1(Y) -> Out1/1
  In3/1 -> [beta]
  In4/1 -> [qbar]
  In5/1 -> [V]
  In6/1 -> [Aileron_L]
  Embedded MATLAB Function1/2(L) -> Out2/1
  In7/1 -> [Aileron_R]
  In8/1 -> [CLw]
  In9/1 -> [CLb]
  In10/1 -> Embedded MATLAB Function1/19(p)
  Embedded MATLAB Function1/3(N) -> Out3/1
  In11/1 -> Embedded MATLAB Function1/20(r)
  In13/1 -> Get_Lr_0_f/1(In1)
  In12/1 -> Embedded MATLAB Function1/21(Rudder)
  get_n_xi/1(Out1) -> Embedded MATLAB Function1/22(Nxi)
  In14/1 -> Embedded MATLAB Function/27(CD0w)
  In15/1 -> Embedded MATLAB Function/28(DelCDi_flap)
  In16/1 -> Embedded MATLAB Function/29(DelCD0_flap)
  In17/1 -> slipstream effects/5(Xp)
  In18/1 -> slipstream effects/6(deu_dap)
  Constant2/1 -> slipstream effects/8(Yv_n)
  Constant7/1 -> slipstream effects/9(Nv_n)
  [qbar] -> slipstream effects/10(qbar)
  Constant13/1 -> slipstream effects/11(D)
  slipstream effects/1(Yv_ns) -> Embedded MATLAB Function/16(Yv_n)
  slipstream effects/5(Nv_ns) -> Embedded MATLAB Function/21(Nv_n)
  In19/1 -> slipstream effects/7(DCLw)
  slipstream effects/2(Lv_s) -> [Lv_slip]
  [Lv_slip] -> Add1/2
  Embedded MATLAB Function/5(Lv) -> Add1/1
  Add1/1 -> Embedded MATLAB Function1/11(Lv)
  slipstream effects/3(Lp_s) -> [Lp_slip]
  [Lp_slip] -> Add2/2
  Embedded MATLAB Function/6(Lp) -> Add2/1
  Add2/1 -> Embedded MATLAB Function1/12(Lp)
  slipstream effects/4(Lr_s) -> [Lr_slip]
  [Lr_slip] -> Add3/2
  Embedded MATLAB Function/7(Lr) -> Add3/1
  Add3/1 -> Embedded MATLAB Function1/13(Lr)
  Constant14/1 -> slipstream effects/2(Xp_dash)
  Constant15/1 -> Demux/1
  Demux/1 -> slipstream effects/3(xp)
  Demux/2 -> slipstream effects/4(yp)
  Demux/3 -> Terminator/1

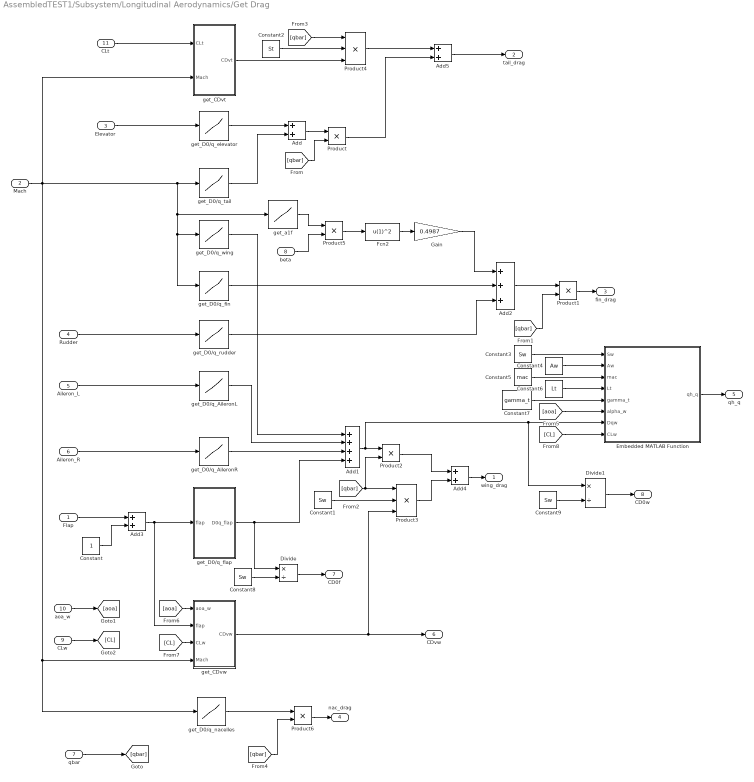
== system AssembledTEST1/Subsystem/Longitudinal Aerodynamics/Get Drag ==
  Flap : Inport
  Mach : Inport  Port=2
  Elevator : Inport  Port=3
  Rudder : Inport  Port=4
  Aileron_L : Inport  Port=5
  Aileron_R : Inport  Port=6
  qbar : Inport  Port=7
  beta : Inport  Port=8
  CLw : Inport  Port=9
  aoa_w : Inport  Port=10
  CLt : Inport  Port=11
  Add{,3..5} (4 alike) : Sum
  Add1 : Sum  Inputs=++++
  Add2 : Sum  Inputs=+++
  Constant : Constant
  Constant{1,3,8..9} (4 alike) : Constant  Value=Sw
  Constant2 : Constant  Value=St
  Constant4 : Constant  Value=Aw
  Constant5 : Constant  Value=mac
  Constant6 : Constant  Value=Lt
  Constant7 : Constant  Value=gamma_t
  Divide : Product  Inputs=*/
  Divide1 : Product  Inputs=*/
  Embedded MATLAB Function : MATLAB Function  TreatAsAtomicUnit=on
  Fcn2 : Fcn  Expr=u(1)^2
  Gain : Gain  Gain=0.4987
  Product{,1..2,5..6} (5 alike) : Product  RndMeth=Zero
  Product3 : Product  Inputs=3  RndMeth=Zero
  Product4 : Product  Inputs=3  RndMeth=Zero
  get_CDvt : Subsystem
  get_CDvw : Subsystem
  get_D0/q_AileronL : Lookup  InputValues=cdrag_data(:,1)  Table=cdrag_data(:,4)
  get_D0/q_AileronR : Lookup  InputValues=cdrag_data(:,1)  Table=cdrag_data(:,4)
  get_D0/q_elevator : Lookup  InputValues=cdrag_data(:,1)  Table=cdrag_data(:,2)
  get_D0/q_fin : Lookup  InputValues=pdrag_data(:,1)  Table=pdrag_data(:,5)
  get_D0/q_flap : Subsystem
  get_D0/q_nacelles : Lookup  InputValues=pdrag_data(:,1)  Table=pdrag_data(:,6)
  get_D0/q_rudder : Lookup  InputValues=cdrag_data(:,1)  Table=cdrag_data(:,3)
  get_D0/q_tail : Lookup  InputValues=pdrag_data(:,1)  Table=pdrag_data(:,4)
  get_D0/q_wing : Lookup  InputValues=pdrag_data(:,1)  Table=pdrag_data(:,2)
  get_a1f : Lookup  InputValues=sideforce_data(:,1)  Table=sideforce_data(:,3)
  wing_drag : Outport
  tail_drag : Outport  Port=2
  fin_drag : Outport  Port=3
  nac_drag : Outport  Port=4
  qh_q : Outport  Port=5
  CDvw : Outport  Port=6
  CD0f : Outport  Port=7
  CD0w : Outport  Port=8
  wires:
  Mach/1 -> get_D0/q_tail/1, get_D0/q_wing/1, get_D0/q_fin/1, get_a1f/1, get_CDvt/2(Mach), get_CDvw/4(Mach), get_D0/q_nacelles/1
  Elevator/1 -> get_D0/q_elevator/1
  Rudder/1 -> get_D0/q_rudder/1
  Aileron_L/1 -> get_D0/q_AileronL/1
  Aileron_R/1 -> get_D0/q_AileronR/1
  get_D0/q_elevator/1 -> Add/1
  get_D0/q_tail/1 -> Add/2
  get_D0/q_wing/1 -> Add1/1
  get_D0/q_AileronL/1 -> Add1/2
  get_D0/q_AileronR/1 -> Add1/3
  Flap/1 -> Add3/1
  Constant/1 -> Add3/2
  Add3/1 -> get_D0/q_flap/1(flap), get_CDvw/2(flap)
  get_D0/q_flap/1(D0q_flap) -> Add1/4, Divide/1
  qbar/1 -> [qbar]
  Add/1 -> Product/1
  [qbar] -> Product/2
  [qbar] -> Product1/2
  Add2/1 -> Product1/1
  [qbar] -> Product3/1, Product2/2
  Add1/1 -> Product2/1, Embedded MATLAB Function/7(Dqw), Divide1/1
  CLt/1 -> get_CDvt/1(CLt)
  Constant1/1 -> Product3/2
  get_CDvw/1(CDvw) -> Product3/3, CDvw/1
  Product2/1 -> Add4/1
  Product3/1 -> Add4/2
  Add4/1 -> wing_drag/1
  [qbar] -> Product4/1
  Constant2/1 -> Product4/2
  Add5/1 -> tail_drag/1
  get_CDvt/1(CDvt) -> Product4/3
  Product4/1 -> Add5/1
  Product/1 -> Add5/2
  get_D0/q_fin/1 -> Add2/2
  get_a1f/1 -> Product5/1
  beta/1 -> Product5/2
  Product5/1 -> Fcn2/1
  Fcn2/1 -> Gain/1
  Gain/1 -> Add2/1
  get_D0/q_rudder/1 -> Add2/3
  Product1/1 -> fin_drag/1
  [qbar] -> Product6/2
  get_D0/q_nacelles/1 -> Product6/1
  Product6/1 -> nac_drag/1
  aoa_w/1 -> [aoa]
  [aoa] -> Embedded MATLAB Function/6(alpha_w)
  CLw/1 -> [CL]
  [aoa] -> get_CDvw/1(aoa_w)
  [CL] -> get_CDvw/3(CLw)
  [CL] -> Embedded MATLAB Function/8(CLw)
  Constant3/1 -> Embedded MATLAB Function/1(Sw)
  Constant4/1 -> Embedded MATLAB Function/2(Aw)
  Constant5/1 -> Embedded MATLAB Function/3(mac)
  Constant6/1 -> Embedded MATLAB Function/4(Lt)
  Constant7/1 -> Embedded MATLAB Function/5(gamma_t)
  Embedded MATLAB Function/1(qh_q) -> qh_q/1
  Divide/1 -> CD0f/1
  Constant8/1 -> Divide/2
  Divide1/1 -> CD0w/1
  Constant9/1 -> Divide1/2

== system AssembledTEST1/Subsystem/Longitudinal Aerodynamics/Get Fin XZM ==
  In2 : Inport
  In1 : Inport  Port=2
  Bus Selector : BusSelector  OutputSignals=alpha_b
  Constant : Constant  Value=xacf
  Constant1 : Constant  Value=zacf
  Get XZM : Subsystem
      mask Display:
      | port_label('input',1,'lift [N]')
      | port_label('input',2,'drag [N]')
      | port_label('input',3,'\alpha [rad]','texmode','on')
      | port_label('input',4,'M_0 [Nm]','texmode','on')
      | port_label('input',5,'x_{ac} [m]','texmode','on')
      | port_label('input',6,'z_{ac} [m]','texmode','on')
      | port_label('output',1,'X [N]')
      | port_label('output',2,'Z [N]')
      | port_label('output',3,'M [Nm]')
  Ground : Ground
  Out1 : Outport
  Out2 : Outport  Port=2
  Out3 : Outport  Port=3
  wires:
  Ground/1 -> Get XZM/1(L), Get XZM/4(M0)
  Get XZM/1(X) -> Out1/1
  In1/1 -> Get XZM/2(D)
  Get XZM/2(Z) -> Out2/1
  Get XZM/3(M) -> Out3/1
  Constant1/1 -> Get XZM/6(z)
  Constant/1 -> Get XZM/5(x)
  In2/1 -> Bus Selector/1
  Bus Selector/1 -> Get XZM/3(alpha)  "<alpha_b>"

== system AssembledTEST1/Subsystem/Longitudinal Aerodynamics/Get Fuselage XZM ==
  Mach : Inport
  Flap : Inport  Port=2
  aoa : Inport  Port=3
  qbar : Inport  Port=4
  q : Inport  Port=5
  Add : Sum
  Constant : Constant  Value=Sw
  Constant1 : Constant  Value=mac
  Constant2 : Constant  Value=Sref
  Constant3 : Constant  Value=DCM0b
  Constant4 : Constant  Value=df
  Embedded MATLAB Function : MATLAB Function  TreatAsAtomicUnit=on
  Gain : Gain  Gain=R2D
  Subsystem : Subsystem
      mask Display:
      | port_label('output',1,'(C_{m\alpha})_{f(\epsilon)}','texmode','on')
      | port_label('input',1,'Flap')
      | port_label('input',2,'Mach')
  get_CM : Lookup  InputValues=[-5:5]  Table=tanh([-5:5])
  get_CN : Lookup  InputValues=[-5:5]  Table=tanh([-5:5])
  get_D0/q : Lookup  InputValues=pdrag_data(:,1)  Table=pdrag_data(:,3)
  get_Mqb : Lookup  InputValues=fus_data(:,1)  Table=fus_data(:,2)
  Xfus : Outport
  Zfus : Outport  Port=2
  Mfus : Outport  Port=3
  wires:
  Mach/1 -> get_D0/q/1, get_Mqb/1, Subsystem/2(In1)
  Flap/1 -> Subsystem/1(In2)
  Embedded MATLAB Function/1(X) -> Xfus/1
  Embedded MATLAB Function/2(Z) -> Zfus/1
  Embedded MATLAB Function/3(M) -> Mfus/1
  get_D0/q/1 -> Embedded MATLAB Function/1(Dq)
  get_Mqb/1 -> Embedded MATLAB Function/2(Mq)
  qbar/1 -> Embedded MATLAB Function/5(qbar)
  q/1 -> Embedded MATLAB Function/6(q)
  Constant/1 -> Embedded MATLAB Function/9(Sw)
  Constant1/1 -> Embedded MATLAB Function/10(mac)
  Add/1 -> Embedded MATLAB Function/11(CM0)
  Constant3/1 -> Add/1
  Subsystem/1(Out1) -> Add/2
  Gain/1 -> get_CN/1, get_CM/1
  aoa/1 -> Gain/1
  get_CN/1 -> Embedded MATLAB Function/3(CN)
  get_CM/1 -> Embedded MATLAB Function/4(CM)
  Constant2/1 -> Embedded MATLAB Function/7(Sref)
  Constant4/1 -> Embedded MATLAB Function/8(df)

== system AssembledTEST1/Subsystem/Longitudinal Aerodynamics/Get Nacelles XZM ==
  In2 : Inport
  In1 : Inport  Port=2
  Bus Selector : BusSelector  OutputSignals=alpha_b,q_bar,Flap,Mach
  Constant : Constant  Value=xacn
  Constant1 : Constant  Value=zacn
  Constant2 : Constant  Value=0
  Constant6 : Constant  Value=mac
  Constant7 : Constant  Value=Sw
  Get XZM : Subsystem
      mask Display:
      | port_label('input',1,'lift [N]')
      | port_label('input',2,'drag [N]')
      | port_label('input',3,'\alpha [rad]','texmode','on')
      | port_label('input',4,'M [Nm]','texmode','on')
      | port_label('input',5,'x_{ac} [m]','texmode','on')
      | port_label('input',6,'z_{ac} [m]','texmode','on')
      | port_label('output',1,'X [N]')
      | port_label('output',2,'Z [N]')
      | port_label('output',3,'M [Nm]')
  Product7 : Product  Inputs=5  RndMeth=Zero
  Subsystem : Subsystem
      mask Display:
      | port_label('output',1,'(C_{m\alpha})_{n(\epsilon)}','texmode','on')
      | port_label('input',1,'Flap')
      | port_label('input',2,'Mach')
  Out1 : Outport
  Out2 : Outport  Port=2
  Out3 : Outport  Port=3
  wires:
  Get XZM/1(X) -> Out1/1
  In1/1 -> Get XZM/2(D)
  Get XZM/2(Z) -> Out2/1
  Get XZM/3(M) -> Out3/1
  Constant1/1 -> Get XZM/6(z)
  Constant/1 -> Get XZM/5(x)
  In2/1 -> Bus Selector/1
  Bus Selector/1 -> Get XZM/3(alpha), Product7/1  "<alpha_b>"
  Constant6/1 -> Product7/2
  Constant7/1 -> Product7/3
  Constant2/1 -> Get XZM/1(L)
  Bus Selector/2 -> Product7/4  "<q_bar>"
  Bus Selector/3 -> Subsystem/1(In2)  "<Flap>"
  Bus Selector/4 -> Subsystem/2(In1)  "<Mach>"
  Subsystem/1(Out1) -> Product7/5
  Product7/1 -> Get XZM/4(M0)

== system AssembledTEST1/Subsystem/Longitudinal Aerodynamics/Get Tail XZM ==
  In1 : Inport
  In2 : Inport  Port=2
  In3 : Inport  Port=3
  In4 : Inport  Port=4
  In5 : Inport  Port=5
  Bus Selector : BusSelector  OutputSignals=Mach,q_bar,Elevator
  Constant1 : Constant  Value=-0.652
  Constant13 : Constant  Value=zact
  Constant2 : Constant  Value=Sw
  Constant3 : Constant  Value=mac
  Get XZM : Subsystem
      mask Display:
      | port_label('input',1,'lift [N]')
      | port_label('input',2,'drag [N]')
      | port_label('input',3,'\alpha [rad]','texmode','on')
      | port_label('input',4,'M_0 [Nm]','texmode','on')
      | port_label('input',5,'x_{ac} [m]','texmode','on')
      | port_label('input',6,'z_{ac} [m]','texmode','on')
      | port_label('output',1,'X [N]')
      | port_label('output',2,'Z [N]')
      | port_label('output',3,'M [Nm]')
  Product1 : Product  Inputs=6  RndMeth=Zero
  get kf : Lookup  InputValues=tail_data(:,1)  Table=tail_data(:,6)
  Out1 : Outport
  Out2 : Outport  Port=2
  Out3 : Outport  Port=3
  wires:
  Constant13/1 -> Get XZM/6(z)
  In1/1 -> Get XZM/1(L)
  Get XZM/1(X) -> Out1/1
  In2/1 -> Get XZM/2(D)
  In3/1 -> Get XZM/3(alpha)
  Get XZM/2(Z) -> Out2/1
  In5/1 -> Get XZM/5(x)
  Get XZM/3(M) -> Out3/1
  In4/1 -> Bus Selector/1
  Bus Selector/1 -> get kf/1  "<Mach>"
  get kf/1 -> Product1/1
  Bus Selector/2 -> Product1/2  "<q_bar>"
  Bus Selector/3 -> Product1/3  "<Elevator>"
  Constant1/1 -> Product1/4
  Constant2/1 -> Product1/5
  Constant3/1 -> Product1/6
  Product1/1 -> Get XZM/4(M0)
